simulink model "UAM_FlightMode"  (R2024b)
settings: Solver=FixedStepAuto  StartTime=0.0  StopTime=10.0  RelTol=1e-3
model workspace: external: MAT-File C:\Users\admin\Desktop\onboard-flight-control-software-ver1.1\data\stateBus.mat (data not in the file)
undefined symbols (not defined in the file): control, FSState, Vt, zGround
libraries: uavalgslib x6, simulink x1
settings Model: DataDictionary=UAM_data.sldd  Creator=admin  LastModifiedBy=admin
settings OptimizationCC: DefaultParameterBehavior=Inlined  EnhancedBackFolding=on  PassReuseOutputArgsAs=Individual arguments  ZeroExternalMemoryAtStartup=off  ZeroInternalMemoryAtStartup=off  OptimizeBlockOrder=speed  DifferentSizesBufferReuse=on  OptimizationCustomize=off  EfficientTunableParamExpr=on
settings DebuggingCC: ParameterTunabilityLossMsg=error
settings HardwareCC: ProdBitPerLong=64  ProdLargestAtomicInteger=LongLong  ProdLargestAtomicFloat=Double  ProdLongLongMode=on  ProdHWDeviceType=ARM Compatible->ARM Cortex-A (64-bit)
settings SFSimCC: MATLABDynamicMemAlloc=off
settings RTWCC: Description=Embedded Coder  SystemTargetFile=ert.tlc  TemplateMakefile=ert_default_tmf  Toolchain=Linaro AArch64 Linux v6.3.1
settings CodeAppCC: ForceParamTrailComments=on  IgnoreCustomStorageClasses=off  OperatorAnnotations=on  SimulinkDataObjDesc=on  SFDataObjDesc=on  CustomSymbolStrGlobalVar=MODE_$N$M  CustomSymbolStrType=MODE_$N$M_T  CustomSymbolStrField=MODE_$N$M  CustomSymbolStrFcn=MODE_$N$M$F  CustomSymbolStrBlkIO=MODE_rtb_$N$M  CustomSymbolStrTmpVar=MODE_tmp_$N$M  CustomSymbolStrMacro=MODE_$N$M_MACRO  InsertBlockDesc=on
settings ERTTargetCC: TargetLangStandard=C99 (ISO)  GenerateSampleERTMain=on  ERTCustomFileTemplate=example_file_process.tlc

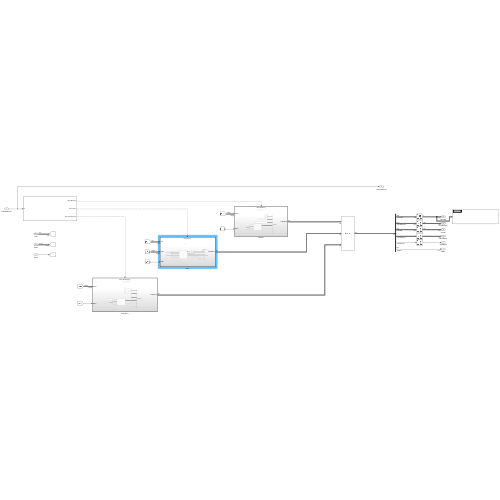
[thumbnail: Simulink's stored preview of the top-level diagram]
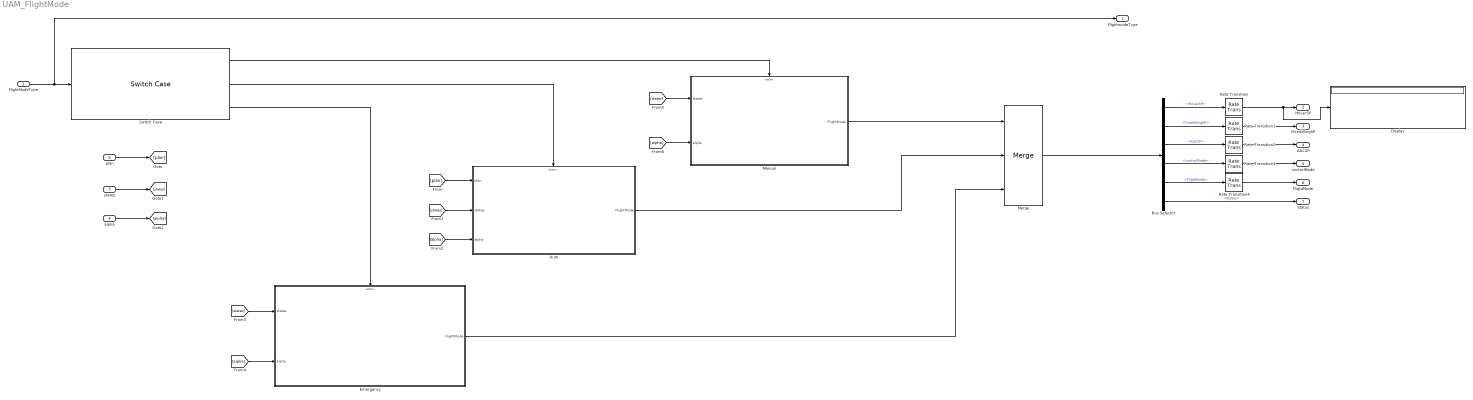
== system UAM_FlightMode ==
  FlightModeType : Inport
  plan : Inport  Port=2  OutDataTypeStr=Bus: plan
  states : Inport  Port=3  OutDataTypeStr=Bus: states
  alpha : Inport  Port=4
  Auto : Subsystem  TreatAsAtomicUnit=on
  Bus Selector : BusSelector  OutputSignals=HoverSP,FixedWingSP,AACSP,controlMode,FlightMode,Status
  Display : Display
  Emergency : Subsystem  TreatAsAtomicUnit=on
  Manual : Subsystem  TreatAsAtomicUnit=on
  Merge : Merge  Inputs=3
  Rate Transition{,1..4} (5 alike) : RateTransition
  Switch Case : SwitchCase  CaseConditions={FlightModeType.Manual, FlightModeType.Auto, FlightModeType.Emergecny}  ShowDefaultCase=off
  FlightmodeType : Outport  OutDataTypeStr=Enum: FlightModeType
  HoverSP : Outport  Port=2  OutDataTypeStr=Bus: HoverSPBus
  FixedWingSP : Outport  Port=3  OutDataTypeStr=Bus: FixedWingCommandBus
  AACSP : Outport  Port=4  OutDataTypeStr=Bus: AAC
  controlMode : Outport  Port=5  OutDataTypeStr=Bus: controlMode
  FlightMode : Outport  Port=6
  Status : Outport  Port=7
  wires:
  FlightModeType/1 -> FlightmodeType/1, Switch Case/1
  plan/1 -> [plan]
  states/1 -> [states]
  [states] -> Auto/2(states)
  [alpha] -> Auto/3(alpha)
  alpha/1 -> [alpha]
  [plan] -> Auto/1(plan)
  Switch Case/2 -> Auto/Action
  Switch Case/1 -> Manual/Action
  Switch Case/3 -> Emergency/Action
  [alpha] -> Emergency/2(alpha)
  [states] -> Emergency/1(states)
  [alpha] -> Manual/2(alpha)
  [states] -> Manual/1(states)
  Manual/1(FlightMode) -> Merge/1
  Bus Selector/4 -> Rate Transition3/1  "<controlMode>"
  Rate Transition1/1 -> FixedWingSP/1
  Bus Selector/5 -> Rate Transition4/1  "<FlightMode>"
  Rate Transition3/1 -> controlMode/1
  Bus Selector/1 -> Rate Transition/1  "<HoverSP>"
  Bus Selector/3 -> Rate Transition2/1  "<AACSP>"
  Rate Transition/1 -> Display/1, HoverSP/1
  Rate Transition4/1 -> FlightMode/1
  Bus Selector/2 -> Rate Transition1/1  "<FixedWingSP>"
  Rate Transition2/1 -> AACSP/1
  Bus Selector/6 -> Status/1  "<Status>"
  Merge/1 -> Bus Selector/1
  Auto/1(FlightMode) -> Merge/2
  Emergency/1(FlightMode) -> Merge/3

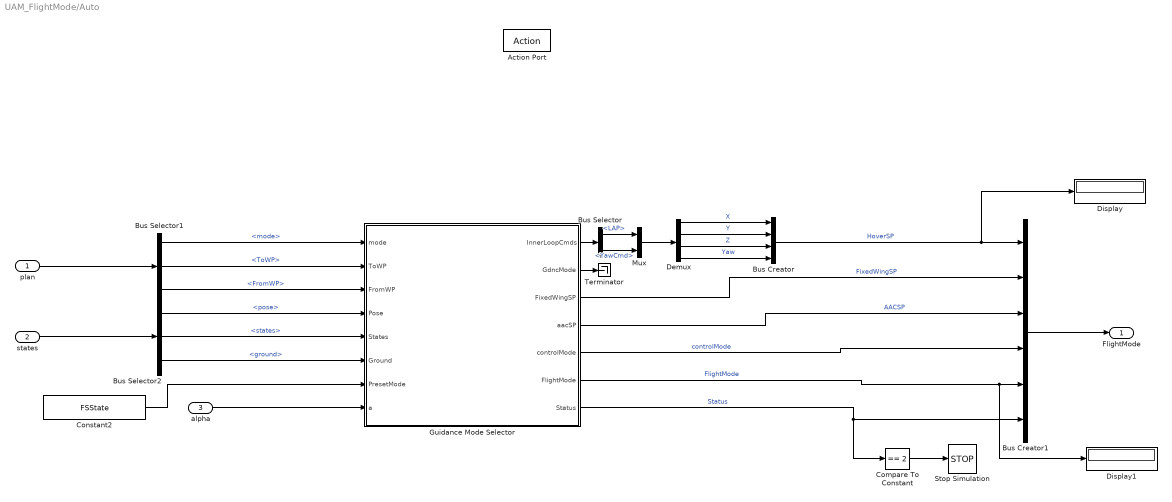
== system UAM_FlightMode/Auto ==
  plan : Inport  OutDataTypeStr=Bus: plan
  states : Inport  Port=2  OutDataTypeStr=Bus: states
  alpha : Inport  Port=3
  Action Port : ActionPort  ActionPortLabel=case [ Auto ]:
  Bus Creator : BusCreator  Inputs=4  OutDataTypeStr=Bus: HoverSPBus
      settings: InheritFromInputs=off
  Bus Creator1 : BusCreator  Inputs=6  OutDataTypeStr=Bus: flightmode
  Bus Selector : BusSelector  OutputSignals=LAP,YawCmd
  Bus Selector1 : BusSelector  OutputSignals=mode,ToWP,FromWP
  Bus Selector2 : BusSelector  OutputSignals=pose,states,ground
  Compare To Constant : simulink/Logic and Bit Operations/Compare To Constant  relop===  const=2  OutDataTypeStr=boolean
  Constant2 : Constant  Value=FSState
  Demux : Demux
  Display : Display
  Display1 : Display
  Guidance Mode Selector : Stateflow chart  TreatAsAtomicUnit=on
      settings: PortSchema="{\"entries\":[{\"content\":{\"sides\":[{\"content\":{\"connectorIds\":[\"In1\",\"In2\",\"In3\",\"In4\",\"In5\",\"In7\",\"In6\",\"In8\"]},\"type\":\"ConnectorPlacement.EquallySpacedRectSide\",\"uuid\":\"a9cfd0e2-196c-422d-b359-9161a47768c9\"},{\"content\":{\"connectorIds\":[\"Out7\",\"Out2\",\"Out4\",\"Out3\",\"Out5\",\"Out6\",\"Out1\"],\"side\":\"RIGHT\"},\"type\":\"ConnectorPlacement.EquallySpacedRectSide\",\"uuid\":\"4fed41ae-e7cf-4de3-8bdb-9e24e7d8b079\"},{\"content\":{\"side\":\"TOP\"},\"type\":\"ConnectorPlacement.EquallySpacedRectSide\",\"uuid\":\"2d49ff20-2f63-498d-ac9d-820eae01f794\"},{\"content\":{\"side\":\"BOTTOM\"},\"type\":\"ConnectorPlacement.EquallySpacedRectSide\",\"uuid\":\"da24ee44-6e15-4e50-9b36-ff21cb47946d\"}]},\"type\":\"ConnectorPlacement.EquallySpacedConnector\",\"uuid\":\"88d403f4-ad96-40f9-9697-84906f26a8bf\"}],\"packageUris\":[\"http://schema.mathworks.com/mf0/Connector/R2020b\"],\"version\":\"1.0\"}"
  Mux : Mux  Inputs=2
  Stop Simulation : Stop
  Terminator : Terminator
  FlightMode : Outport  OutDataTypeStr=Bus: flightmode
  wires:
  Bus Selector1/1 -> Guidance Mode Selector/1(mode)  "<mode>"
  Guidance Mode Selector/6(FlightMode) -> Display1/1, Bus Creator1/5  "FlightMode"
  Bus Selector1/3 -> Guidance Mode Selector/3(FromWP)  "<FromWP>"
  Bus Selector2/3 -> Guidance Mode Selector/7(Ground)  "<ground>"
  Bus Selector/1 -> Mux/1  "<LAP>"
  Guidance Mode Selector/5(controlMode) -> Bus Creator1/4  "controlMode"
  Guidance Mode Selector/3(aacSP) -> Bus Creator1/3  "AACSP"
  alpha/1 -> Guidance Mode Selector/8(a)
  Guidance Mode Selector/7(InnerLoopCmds) -> Bus Selector/1
  Guidance Mode Selector/2(GdncMode) -> Terminator/1
  Bus Selector/2 -> Mux/2  "<YawCmd>"
  Compare To Constant/1 -> Stop Simulation/1
  Bus Selector2/2 -> Guidance Mode Selector/5(States)  "<states>"
  Mux/1 -> Demux/1
  plan/1 -> Bus Selector1/1
  states/1 -> Bus Selector2/1
  Bus Selector2/1 -> Guidance Mode Selector/4(Pose)  "<pose>"
  Guidance Mode Selector/1(Status) -> Compare To Constant/1, Bus Creator1/6  "Status"
  Guidance Mode Selector/4(FixedWingSP) -> Bus Creator1/2  "FixedWingSP"
  Constant2/1 -> Guidance Mode Selector/6(PresetMode)
  Bus Selector1/2 -> Guidance Mode Selector/2(ToWP)  "<ToWP>"
  Bus Creator1/1 -> FlightMode/1
  Demux/1 -> Bus Creator/1  "X"
  Demux/2 -> Bus Creator/2  "Y"
  Demux/3 -> Bus Creator/3  "Z"
  Demux/4 -> Bus Creator/4  "Yaw"
  Bus Creator/1 -> Display/1, Bus Creator1/1  "HoverSP"

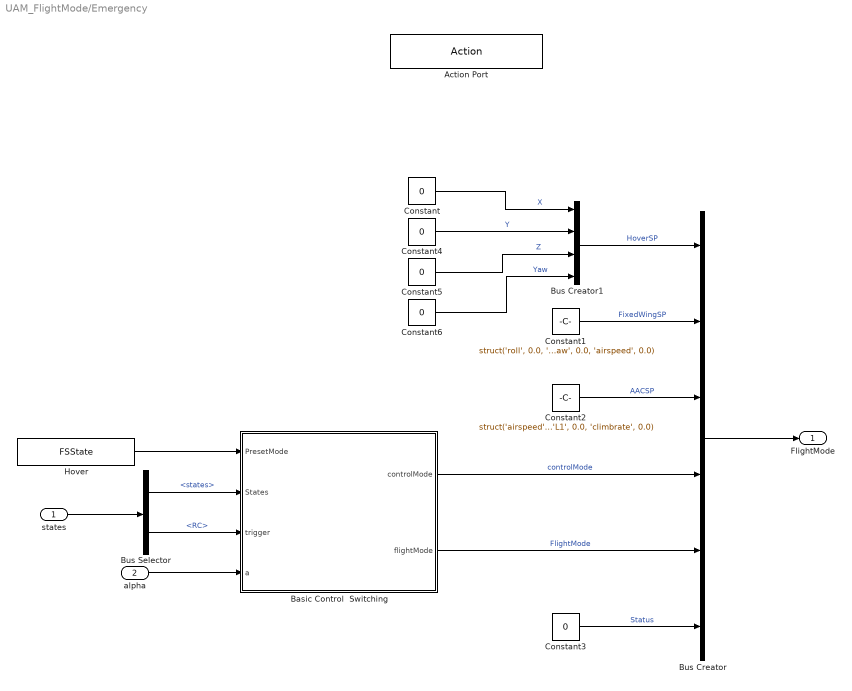
== system UAM_FlightMode/Emergency ==
  states : Inport  OutDataTypeStr=Bus: states
  alpha : Inport  Port=2
  Action Port : ActionPort  ActionPortLabel=case [ Emergecny ]:
  Basic Control  Switching : Stateflow chart  TreatAsAtomicUnit=on
  Bus Creator : BusCreator  Inputs=6  OutDataTypeStr=Bus: flightmode
      settings: InheritFromInputs=off
  Bus Creator1 : BusCreator  Inputs=4  OutDataTypeStr=Bus: HoverSPBus
  Bus Selector : BusSelector  OutputSignals=states,states.RC
  Constant{,4..6} (4 alike) : Constant  Value=0
  Constant1 : Constant  Value=struct('roll', 0.0, 'pitch', 0.0, 'yaw', 0.0, 'airspeed', 0.0)  VectorParams1D=off  OutDataTypeStr=Bus: FixedWingCommandBus
  Constant2 : Constant  Value=struct('airspeed', 0.0, 'altitude', 0.0, 'course', 0.0, 'L1', 0.0, 'climbrate', 0.0)  VectorParams1D=off  OutDataTypeStr=Bus: AAC
  Constant3 : Constant  Value=0  OutDataTypeStr=uint8
  Hover : Constant  Value=FSState
  FlightMode : Outport  OutDataTypeStr=Bus: flightmode
  wires:
  Constant/1 -> Bus Creator1/1  "X"
  Constant5/1 -> Bus Creator1/3  "Z"
  Constant4/1 -> Bus Creator1/2  "Y"
  Basic Control  Switching/2(flightMode) -> Bus Creator/5  "FlightMode"
  Basic Control  Switching/1(controlMode) -> Bus Creator/4  "controlMode"
  Hover/1 -> Basic Control  Switching/1(PresetMode)
  Constant3/1 -> Bus Creator/6  "Status"
  Bus Selector/2 -> Basic Control  Switching/3(trigger)  "<RC>"
  Bus Selector/1 -> Basic Control  Switching/2(States)  "<states>"
  Constant2/1 -> Bus Creator/3  "AACSP"
  alpha/1 -> Basic Control  Switching/4(a)
  Bus Creator1/1 -> Bus Creator/1  "HoverSP"
  states/1 -> Bus Selector/1
  Constant1/1 -> Bus Creator/2  "FixedWingSP"
  Constant6/1 -> Bus Creator1/4  "Yaw"
  Bus Creator/1 -> FlightMode/1

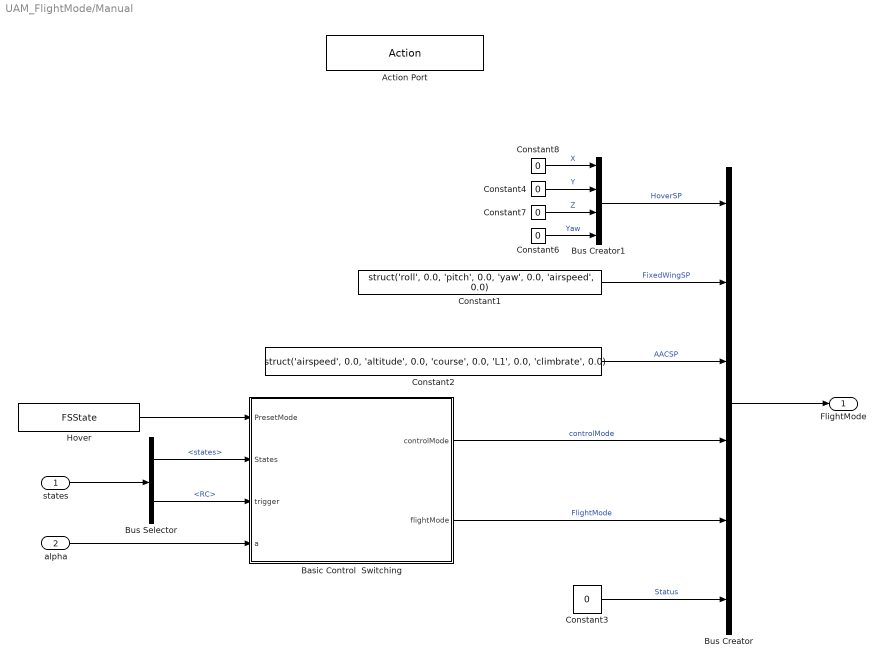
== system UAM_FlightMode/Manual ==
  states : Inport  OutDataTypeStr=Bus: states
  alpha : Inport  Port=2
  Action Port : ActionPort  ActionPortLabel=case [ Manual ]:
  Basic Control  Switching : Stateflow chart  TreatAsAtomicUnit=on
  Bus Creator : BusCreator  Inputs=6  OutDataTypeStr=Bus: flightmode
      settings: InheritFromInputs=off
  Bus Creator1 : BusCreator  Inputs=4  OutDataTypeStr=Bus: HoverSPBus
  Bus Selector : BusSelector  OutputSignals=states,states.RC
  Constant1 : Constant  Value=struct('roll', 0.0, 'pitch', 0.0, 'yaw', 0.0, 'airspeed', 0.0)  VectorParams1D=off  OutDataTypeStr=Bus: FixedWingCommandBus
  Constant2 : Constant  Value=struct('airspeed', 0.0, 'altitude', 0.0, 'course', 0.0, 'L1', 0.0, 'climbrate', 0.0)  VectorParams1D=off  OutDataTypeStr=Bus: AAC
  Constant3 : Constant  Value=0  OutDataTypeStr=uint8
  Constant{4,6..8} (4 alike) : Constant  Value=0
  Hover : Constant  Value=FSState
  FlightMode : Outport  OutDataTypeStr=Bus: flightmode
  wires:
  states/1 -> Bus Selector/1
  Basic Control  Switching/1(controlMode) -> Bus Creator/4  "controlMode"
  Hover/1 -> Basic Control  Switching/1(PresetMode)
  Basic Control  Switching/2(flightMode) -> Bus Creator/5  "FlightMode"
  Constant3/1 -> Bus Creator/6  "Status"
  Bus Creator/1 -> FlightMode/1
  Bus Creator1/1 -> Bus Creator/1  "HoverSP"
  Constant2/1 -> Bus Creator/3  "AACSP"
  Constant1/1 -> Bus Creator/2  "FixedWingSP"
  alpha/1 -> Basic Control  Switching/4(a)
  Bus Selector/1 -> Basic Control  Switching/2(States)  "<states>"
  Bus Selector/2 -> Basic Control  Switching/3(trigger)  "<RC>"
  Constant6/1 -> Bus Creator1/4  "Yaw"
  Constant7/1 -> Bus Creator1/3  "Z"
  Constant4/1 -> Bus Creator1/2  "Y"
  Constant8/1 -> Bus Creator1/1  "X"

== system UAM_FlightMode/Auto/Guidance Mode Selector/GuidanceLogic.BackTransition ==
  States : Inport  OutDataTypeStr=Bus: GuidanceStates
  Action Port : ActionPort
      settings: CopyFcn=Stateflow.SLINSF.SimulinkMan.removeBlockPreDeleteFcn  PreDeleteFcn=Stateflow.SLINSF.SimulinkMan.unsafePredeleteFcn
  Bus Creator1 : BusCreator  Inputs=3  OutDataTypeStr=Bus: innerLoopCmdsBus  NonVirtualBus=on
  Bus Selector : BusSelector  OutputSignals=Xe
  Constant : Constant  Value=0
  Constant1 : Constant  Value=0
  Constant2 : Constant  Value=0
  Data Type Conversion : DataTypeConversion  OutDataTypeStr=uint8  SaturateOnIntegerOverflow=off  RndMeth=Floor
  Gain : Gain
  Status : Outport
  InnerLoopCmds : Outport  Port=2  OutDataTypeStr=Bus: innerLoopCmdsBus
  wires:
  States/1 -> Bus Selector/1
  Bus Selector/1 -> Gain/1  "<Xe>"
  Bus Creator1/1 -> InnerLoopCmds/1
  Constant1/1 -> Bus Creator1/2  "HeadingCmd"
  Constant2/1 -> Bus Creator1/3  "YawCmd"
  Data Type Conversion/1 -> Status/1
  Gain/1 -> Bus Creator1/1  "LAP"
  Constant/1 -> Data Type Conversion/1

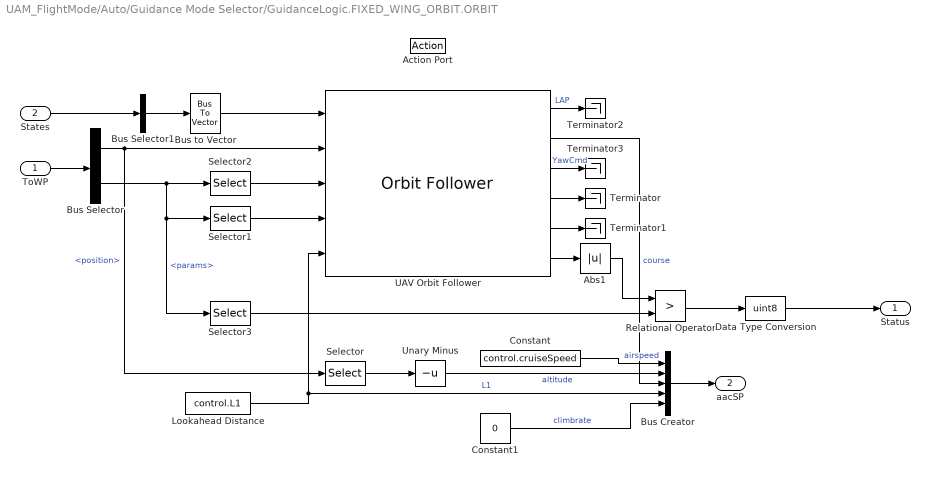
== system UAM_FlightMode/Auto/Guidance Mode Selector/GuidanceLogic.FIXED_WING_ORBIT.ORBIT ==
  ToWP : Inport  OutDataTypeStr=Bus: UAVPathManagerBus
  States : Inport  Port=2
  Action Port : ActionPort
      settings: CopyFcn=Stateflow.SLINSF.SimulinkMan.removeBlockPreDeleteFcn  PreDeleteFcn=Stateflow.SLINSF.SimulinkMan.unsafePredeleteFcn
  Abs1 : Abs  SaturateOnIntegerOverflow=off
  Bus Creator : BusCreator  Inputs=5  OutDataTypeStr=Bus: AAC  NonVirtualBus=on
      settings: InheritFromInputs=off
  Bus Selector : BusSelector  OutputSignals=position,params
  Bus Selector1 : BusSelector  OutputSignals=Xe,course  OutputAsBus=on
  Bus to Vector : BusToVector
  Constant : Constant  Value=control.cruiseSpeed
  Constant1 : Constant  Value=0
  Data Type Conversion : DataTypeConversion  OutDataTypeStr=uint8  SaturateOnIntegerOverflow=off  RndMeth=Floor
  Lookahead Distance : Constant  Value=control.L1  OutDataTypeStr=double
  Relational Operator : RelationalOperator  Operator=>  OutDataTypeStr=boolean  RndMeth=Simplest  InputSameDT=off
  Selector : Selector  InputPortWidth=3  IndexOptions=Index vector (dialog)  Indices=3  OutputSizes=1
  Selector1 : Selector  InputPortWidth=4  IndexOptions=Index vector (dialog)  Indices=2  OutputSizes=1
  Selector2 : Selector  InputPortWidth=4  IndexOptions=Index vector (dialog)  Indices=1  OutputSizes=1
  Selector3 : Selector  InputPortWidth=4  IndexOptions=Index vector (dialog)  Indices=3  OutputSizes=1
  Terminator{,1..3} (4 alike) : Terminator
  UAV Orbit Follower : uavalgslib/Orbit Follower  UAVType=fixed-wing  MinOrbitRadius=control.turningRadius  MinLookaheadDistance=control.L1  ExternalReset=none  ShowCrossTrackErrorOutput=off  ShowNumTurnsOutput=on  SimulateUsing=Code generation
  Unary Minus : UnaryMinus
  Status : Outport
  aacSP : Outport  Port=2
  wires:
  Bus to Vector/1 -> UAV Orbit Follower/1
  Selector2/1 -> UAV Orbit Follower/3
  Bus Selector/1 -> UAV Orbit Follower/2, Selector/1  "<position>"
  ToWP/1 -> Bus Selector/1
  Bus Selector/2 -> Selector1/1, Selector3/1, Selector2/1  "<params>"
  Selector3/1 -> Relational Operator/2
  Relational Operator/1 -> Data Type Conversion/1
  UAV Orbit Follower/4 -> Terminator/1
  UAV Orbit Follower/5 -> Terminator1/1
  Bus Selector1/1 -> Bus to Vector/1
  States/1 -> Bus Selector1/1
  UAV Orbit Follower/1 -> Terminator2/1  "LAP"
  Lookahead Distance/1 -> UAV Orbit Follower/5, Bus Creator/4  "L1"
  Bus Creator/1 -> aacSP/1
  UAV Orbit Follower/2 -> Bus Creator/3  "course"
  Constant/1 -> Bus Creator/1  "airspeed"
  Unary Minus/1 -> Bus Creator/2  "altitude"
  UAV Orbit Follower/3 -> Terminator3/1  "YawCmd"
  Selector/1 -> Unary Minus/1
  UAV Orbit Follower/6 -> Abs1/1
  Abs1/1 -> Relational Operator/1
  Selector1/1 -> UAV Orbit Follower/4
  Constant1/1 -> Bus Creator/5  "climbrate"
  Data Type Conversion/1 -> Status/1

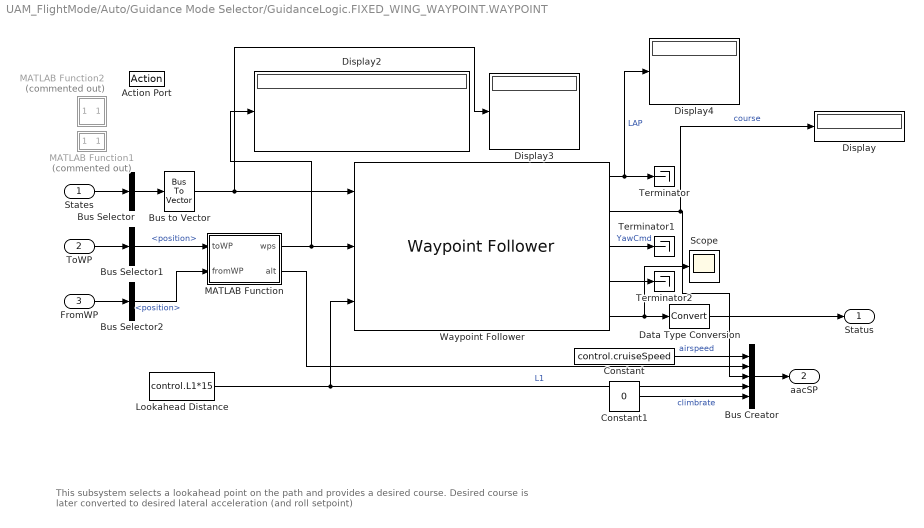
== system UAM_FlightMode/Auto/Guidance Mode Selector/GuidanceLogic.FIXED_WING_WAYPOINT.WAYPOINT ==
  note: This subsystem selects a lookahead point on the path and provides a desired course. Desired course is later converted to desired lateral acceleration (and roll setpoint)
  States : Inport  OutDataTypeStr=Bus: GuidanceStates
  ToWP : Inport  Port=2  OutDataTypeStr=Bus: UAVPathManagerBus
  FromWP : Inport  Port=3  OutDataTypeStr=Bus: UAVPathManagerBus
  Action Port : ActionPort
      settings: CopyFcn=Stateflow.SLINSF.SimulinkMan.removeBlockPreDeleteFcn  PreDeleteFcn=Stateflow.SLINSF.SimulinkMan.unsafePredeleteFcn
  Bus Creator : BusCreator  Inputs=5  OutDataTypeStr=Bus: AAC  NonVirtualBus=on
      settings: InheritFromInputs=off
  Bus Selector : BusSelector  OutputSignals=Xe,course  OutputAsBus=on
  Bus Selector1 : BusSelector  OutputSignals=position
  Bus Selector2 : BusSelector  OutputSignals=position
  Bus to Vector : BusToVector
  Constant : Constant  Value=control.cruiseSpeed
  Constant1 : Constant  Value=0
  Data Type Conversion : DataTypeConversion  SaturateOnIntegerOverflow=off  RndMeth=Floor
  Display{,2..4} (4 alike) : Display
  Lookahead Distance : Constant  Value=control.L1*15  OutDataTypeStr=double
  MATLAB Function : MATLAB Function  TreatAsAtomicUnit=on
  MATLAB Function1 : MATLAB Function  Commented=on  TreatAsAtomicUnit=on
  MATLAB Function2 : MATLAB Function  Commented=on  TreatAsAtomicUnit=on
  Scope : Scope
  Terminator : Terminator
  Terminator1 : Terminator
  Terminator2 : Terminator
  Waypoint Follower : uavalgslib/Waypoint Follower  UAVType=fixed-wing  StartFrom=first  TransitionRadiusSource=internal  TransitionRadius=FWControl.transitionRadius  MinLookaheadDistance=control.L1  HoverAtLastWaypoint=off  YawInput=off  ShowCrossTrackErrorOutput=off  ShowStatusOutput=on  SimulateUsing=Code generation
  Status : Outport
  aacSP : Outport  Port=2
  wires:
  Lookahead Distance/1 -> Waypoint Follower/3, Bus Creator/4  "L1"
  Waypoint Follower/1 -> Display4/1, Terminator/1  "LAP"
  Waypoint Follower/3 -> Terminator1/1  "YawCmd"
  Waypoint Follower/4 -> Terminator2/1
  Constant/1 -> Bus Creator/1  "airspeed"
  States/1 -> Bus Selector/1
  Bus Selector/1 -> Bus to Vector/1
  Waypoint Follower/5 -> Scope/1, Data Type Conversion/1
  Data Type Conversion/1 -> Status/1
  Bus Creator/1 -> aacSP/1
  ToWP/1 -> Bus Selector1/1
  FromWP/1 -> Bus Selector2/1
  Bus Selector1/1 -> MATLAB Function/1(toWP)  "<position>"
  Bus Selector2/1 -> MATLAB Function/2(fromWP)  "<position>"
  MATLAB Function/2(alt) -> Bus Creator/2
  Waypoint Follower/2 -> Display/1, Bus Creator/3  "course"
  Constant1/1 -> Bus Creator/5  "climbrate"
  Bus to Vector/1 -> Display3/1, Waypoint Follower/1
  MATLAB Function/1(wps) -> Display2/1, Waypoint Follower/2

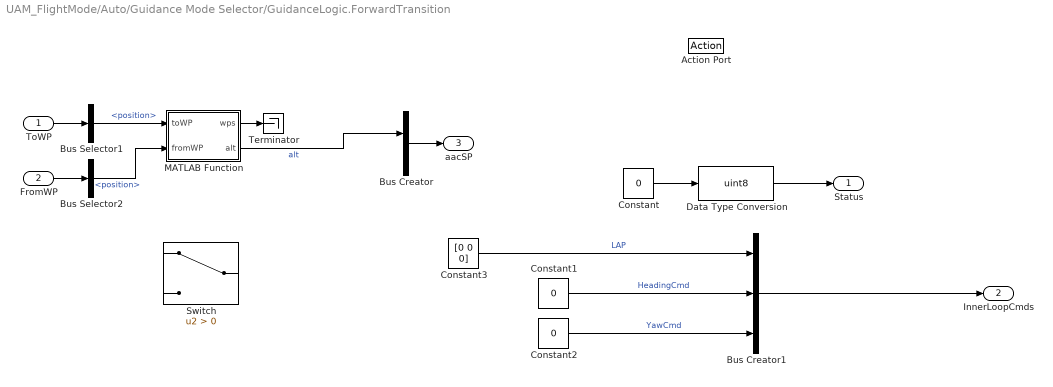
== system UAM_FlightMode/Auto/Guidance Mode Selector/GuidanceLogic.ForwardTransition ==
  ToWP : Inport  OutDataTypeStr=Bus: UAVPathManagerBus
  FromWP : Inport  Port=2  OutDataTypeStr=Bus: UAVPathManagerBus
  Action Port : ActionPort
      settings: CopyFcn=Stateflow.SLINSF.SimulinkMan.removeBlockPreDeleteFcn  PreDeleteFcn=Stateflow.SLINSF.SimulinkMan.unsafePredeleteFcn
  Bus Creator : BusCreator  Inputs=5  OutDataTypeStr=Bus: AAC  NonVirtualBus=on
      settings: InheritFromInputs=off
  Bus Creator1 : BusCreator  Inputs=3  OutDataTypeStr=Bus: innerLoopCmdsBus  NonVirtualBus=on
  Bus Selector1 : BusSelector  OutputSignals=position
  Bus Selector2 : BusSelector  OutputSignals=position
  Constant : Constant  Value=0
  Constant1 : Constant  Value=0
  Constant2 : Constant  Value=0
  Constant3 : Constant  Value=[0 0 0]
  Data Type Conversion : DataTypeConversion  OutDataTypeStr=uint8  SaturateOnIntegerOverflow=off  RndMeth=Floor
  MATLAB Function : MATLAB Function  TreatAsAtomicUnit=on
  Switch : Switch  Criteria=u2 > Threshold  SaturateOnIntegerOverflow=off  InputSameDT=off
  Terminator : Terminator
  Status : Outport
  InnerLoopCmds : Outport  Port=2  OutDataTypeStr=Bus: innerLoopCmdsBus
  aacSP : Outport  Port=3
  wires:
  Bus Creator1/1 -> InnerLoopCmds/1
  Constant1/1 -> Bus Creator1/2  "HeadingCmd"
  Constant2/1 -> Bus Creator1/3  "YawCmd"
  Data Type Conversion/1 -> Status/1
  Constant/1 -> Data Type Conversion/1
  Constant3/1 -> Bus Creator1/1  "LAP"
  FromWP/1 -> Bus Selector2/1
  Bus Selector1/1 -> MATLAB Function/1(toWP)  "<position>"
  Bus Selector2/1 -> MATLAB Function/2(fromWP)  "<position>"
  ToWP/1 -> Bus Selector1/1
  Bus Creator/1 -> aacSP/1
  MATLAB Function/1(wps) -> Terminator/1
  MATLAB Function/2(alt) -> Bus Creator/2  "alt"

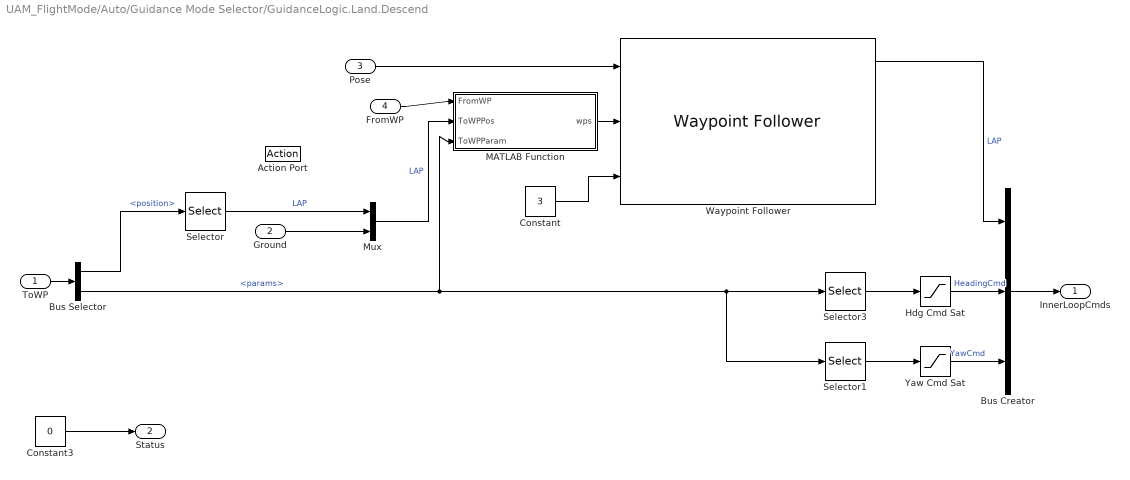
== system UAM_FlightMode/Auto/Guidance Mode Selector/GuidanceLogic.Land.Descend ==
  ToWP : Inport  OutDataTypeStr=Bus: UAVPathManagerBus
  Ground : Inport  Port=2
  Pose : Inport  Port=3
  FromWP : Inport  Port=4  OutDataTypeStr=Bus: UAVPathManagerBus
  Action Port : ActionPort
      settings: CopyFcn=Stateflow.SLINSF.SimulinkMan.removeBlockPreDeleteFcn  PreDeleteFcn=Stateflow.SLINSF.SimulinkMan.unsafePredeleteFcn
  Bus Creator : BusCreator  Inputs=3  OutDataTypeStr=Bus: innerLoopCmdsBus  NonVirtualBus=on
      settings: InheritFromInputs=off
  Bus Selector : BusSelector  OutputSignals=position,params
  Constant : Constant  Value=3
  Constant3 : Constant  Value=0  OutDataTypeStr=uint8
  Hdg Cmd Sat : Saturate  UpperLimit=pi  LowerLimit=-pi
      settings: AttributesFormatString=[%<UpperLimit> %<LowerLimit>]
  MATLAB Function : MATLAB Function  TreatAsAtomicUnit=on
  Mux : Mux  Inputs=2
  Selector : Selector  InputPortWidth=3  IndexOptions=Index vector (dialog)  Indices=[1 2]  OutputSizes=1
  Selector1 : Selector  InputPortWidth=4  IndexOptions=Index vector (dialog)  Indices=4  OutputSizes=1
  Selector3 : Selector  InputPortWidth=4  IndexOptions=Index vector (dialog)  Indices=4  OutputSizes=1
  Waypoint Follower : uavalgslib/Waypoint Follower  UAVType=multirotor  StartFrom=first  TransitionRadiusSource=internal  TransitionRadius=1  MinLookaheadDistance=0.1  HoverAtLastWaypoint=on  YawInput=on  ShowCrossTrackErrorOutput=off  ShowStatusOutput=off  SimulateUsing=Code generation
  Yaw Cmd Sat : Saturate  UpperLimit=pi  LowerLimit=-pi
      settings: AttributesFormatString=[%<UpperLimit> %<LowerLimit>]
  InnerLoopCmds : Outport  OutDataTypeStr=Bus: innerLoopCmdsBus
  Status : Outport  Port=2
  wires:
  Bus Creator/1 -> InnerLoopCmds/1
  Bus Selector/1 -> Selector/1  "<position>"
  Yaw Cmd Sat/1 -> Bus Creator/3  "YawCmd"
  Hdg Cmd Sat/1 -> Bus Creator/2  "HeadingCmd"
  ToWP/1 -> Bus Selector/1
  Selector1/1 -> Yaw Cmd Sat/1
  Selector3/1 -> Hdg Cmd Sat/1
  Selector/1 -> Mux/1  "LAP"
  Bus Selector/2 -> MATLAB Function/3(ToWPParam), Selector1/1, Selector3/1  "<params>"
  Ground/1 -> Mux/2
  Constant3/1 -> Status/1
  Mux/1 -> MATLAB Function/2(ToWPPos)  "LAP"
  FromWP/1 -> MATLAB Function/1(FromWP)
  Pose/1 -> Waypoint Follower/1
  MATLAB Function/1(wps) -> Waypoint Follower/2
  Constant/1 -> Waypoint Follower/3
  Waypoint Follower/1 -> Bus Creator/1  "LAP"

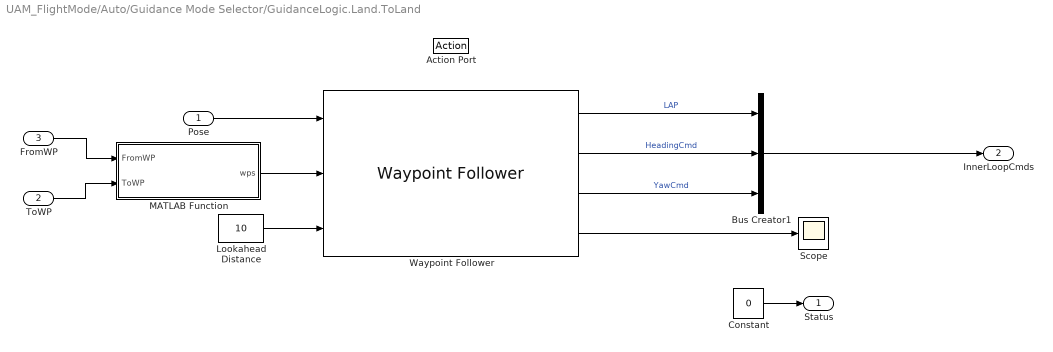
== system UAM_FlightMode/Auto/Guidance Mode Selector/GuidanceLogic.Land.ToLand ==
  Pose : Inport
  ToWP : Inport  Port=2  OutDataTypeStr=Bus: UAVPathManagerBus
  FromWP : Inport  Port=3  OutDataTypeStr=Bus: UAVPathManagerBus
  Action Port : ActionPort
      settings: CopyFcn=Stateflow.SLINSF.SimulinkMan.removeBlockPreDeleteFcn  PreDeleteFcn=Stateflow.SLINSF.SimulinkMan.unsafePredeleteFcn
  Bus Creator1 : BusCreator  Inputs=3  OutDataTypeStr=Bus: innerLoopCmdsBus  NonVirtualBus=on
  Constant : Constant  Value=0  OutDataTypeStr=uint8
  Lookahead Distance : Constant  Value=10  OutDataTypeStr=double
  MATLAB Function : MATLAB Function  TreatAsAtomicUnit=on
  Scope : Scope
  Waypoint Follower : uavalgslib/Waypoint Follower  UAVType=multirotor  StartFrom=first  TransitionRadiusSource=internal  TransitionRadius=1  MinLookaheadDistance=0.1  HoverAtLastWaypoint=on  YawInput=on  ShowCrossTrackErrorOutput=off  ShowStatusOutput=off  SimulateUsing=Code generation
  Status : Outport
  InnerLoopCmds : Outport  Port=2  OutDataTypeStr=Bus: innerLoopCmdsBus
  wires:
  Constant/1 -> Status/1
  MATLAB Function/1(wps) -> Waypoint Follower/2
  Lookahead Distance/1 -> Waypoint Follower/3
  Bus Creator1/1 -> InnerLoopCmds/1
  ToWP/1 -> MATLAB Function/2(ToWP)
  Waypoint Follower/2 -> Bus Creator1/2  "HeadingCmd"
  FromWP/1 -> MATLAB Function/1(FromWP)
  Waypoint Follower/4 -> Scope/1
  Pose/1 -> Waypoint Follower/1
  Waypoint Follower/3 -> Bus Creator1/3  "YawCmd"
  Waypoint Follower/1 -> Bus Creator1/1  "LAP"

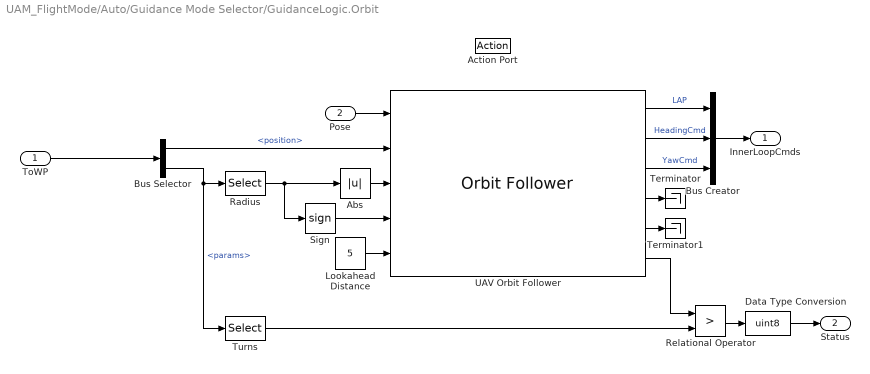
== system UAM_FlightMode/Auto/Guidance Mode Selector/GuidanceLogic.Orbit ==
  ToWP : Inport  OutDataTypeStr=Bus: UAVPathManagerBus
  Pose : Inport  Port=2
  Action Port : ActionPort
      settings: CopyFcn=Stateflow.SLINSF.SimulinkMan.removeBlockPreDeleteFcn  PreDeleteFcn=Stateflow.SLINSF.SimulinkMan.unsafePredeleteFcn
  Abs : Abs  SaturateOnIntegerOverflow=off
  Bus Creator : BusCreator  Inputs=3  OutDataTypeStr=Bus: innerLoopCmdsBus  NonVirtualBus=on
  Bus Selector : BusSelector  OutputSignals=position,params
  Data Type Conversion : DataTypeConversion  OutDataTypeStr=uint8  SaturateOnIntegerOverflow=off  RndMeth=Floor
  Lookahead Distance : Constant  Value=5  OutDataTypeStr=double
  Radius : Selector  InputPortWidth=4  IndexOptions=Index vector (dialog)  Indices=[3]  OutputSizes=1
  Relational Operator : RelationalOperator  Operator=>  OutDataTypeStr=boolean  RndMeth=Simplest  InputSameDT=off
  Sign : Signum  ZeroCross=off
  Terminator : Terminator
  Terminator1 : Terminator
  Turns : Selector  InputPortWidth=4  IndexOptions=Index vector (dialog)  Indices=[1]  OutputSizes=1
  UAV Orbit Follower : uavalgslib/Orbit Follower  UAVType=multirotor  MinOrbitRadius=1  MinLookaheadDistance=0.1  ExternalReset=none  ShowCrossTrackErrorOutput=off  ShowNumTurnsOutput=on  SimulateUsing=Code generation
  InnerLoopCmds : Outport  OutDataTypeStr=Bus: innerLoopCmdsBus
  Status : Outport  Port=2
  wires:
  Pose/1 -> UAV Orbit Follower/1
  Lookahead Distance/1 -> UAV Orbit Follower/5
  Abs/1 -> UAV Orbit Follower/3
  Bus Selector/1 -> UAV Orbit Follower/2  "<position>"
  ToWP/1 -> Bus Selector/1
  Bus Creator/1 -> InnerLoopCmds/1
  UAV Orbit Follower/2 -> Bus Creator/2  "HeadingCmd"
  UAV Orbit Follower/3 -> Bus Creator/3  "YawCmd"
  Bus Selector/2 -> Turns/1, Radius/1  "<params>"
  Radius/1 -> Abs/1, Sign/1
  Sign/1 -> UAV Orbit Follower/4
  Relational Operator/1 -> Data Type Conversion/1
  Turns/1 -> Relational Operator/2
  Data Type Conversion/1 -> Status/1
  UAV Orbit Follower/6 -> Relational Operator/1
  UAV Orbit Follower/4 -> Terminator/1
  UAV Orbit Follower/5 -> Terminator1/1
  UAV Orbit Follower/1 -> Bus Creator/1  "LAP"

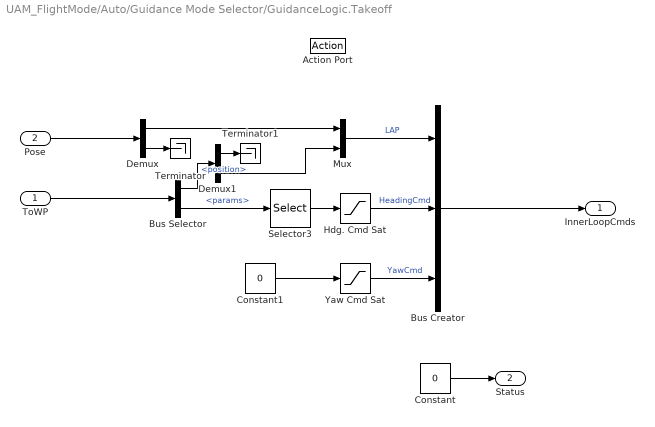
== system UAM_FlightMode/Auto/Guidance Mode Selector/GuidanceLogic.Takeoff ==
  ToWP : Inport  OutDataTypeStr=Bus: UAVPathManagerBus
  Pose : Inport  Port=2
  Action Port : ActionPort
      settings: CopyFcn=Stateflow.SLINSF.SimulinkMan.removeBlockPreDeleteFcn  PreDeleteFcn=Stateflow.SLINSF.SimulinkMan.unsafePredeleteFcn
  Bus Creator : BusCreator  Inputs=3  OutDataTypeStr=Bus: innerLoopCmdsBus  NonVirtualBus=on
      settings: InheritFromInputs=off
  Bus Selector : BusSelector  OutputSignals=position,params
  Constant : Constant  Value=0  OutDataTypeStr=uint8
  Constant1 : Constant  Value=0
  Demux : Demux  Outputs=[2 2]
  Demux1 : Demux  Outputs=[2 1]
  Hdg. Cmd Sat : Saturate  UpperLimit=pi  LowerLimit=-pi
      settings: AttributesFormatString=[%<UpperLimit> %<LowerLimit>]
  Mux : Mux  Inputs=2
  Selector3 : Selector  InputPortWidth=4  IndexOptions=Index vector (dialog)  Indices=4  OutputSizes=1
  Terminator : Terminator
  Terminator1 : Terminator
  Yaw Cmd Sat : Saturate  UpperLimit=pi  LowerLimit=-pi
      settings: AttributesFormatString=[%<UpperLimit> %<LowerLimit>]
  InnerLoopCmds : Outport  OutDataTypeStr=Bus: innerLoopCmdsBus
  Status : Outport  Port=2
  wires:
  Hdg. Cmd Sat/1 -> Bus Creator/2  "HeadingCmd"
  Bus Creator/1 -> InnerLoopCmds/1
  Constant/1 -> Status/1
  Pose/1 -> Demux/1
  Yaw Cmd Sat/1 -> Bus Creator/3  "YawCmd"
  ToWP/1 -> Bus Selector/1
  Bus Selector/2 -> Selector3/1  "<params>"
  Demux/1 -> Mux/1
  Bus Selector/1 -> Demux1/1  "<position>"
  Demux/2 -> Terminator/1
  Demux1/1 -> Terminator1/1
  Selector3/1 -> Hdg. Cmd Sat/1
  Constant1/1 -> Yaw Cmd Sat/1
  Demux1/2 -> Mux/2
  Mux/1 -> Bus Creator/1  "LAP"

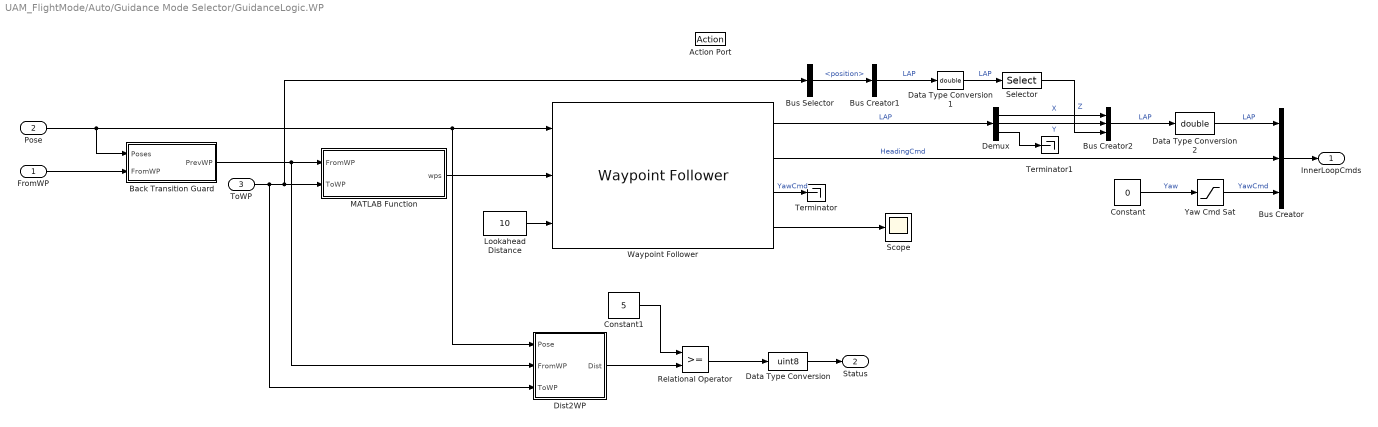
== system UAM_FlightMode/Auto/Guidance Mode Selector/GuidanceLogic.WP ==
  FromWP : Inport  OutDataTypeStr=Bus: UAVPathManagerBus
  Pose : Inport  Port=2
  ToWP : Inport  Port=3  OutDataTypeStr=Bus: UAVPathManagerBus
  Action Port : ActionPort
      settings: CopyFcn=Stateflow.SLINSF.SimulinkMan.removeBlockPreDeleteFcn  PreDeleteFcn=Stateflow.SLINSF.SimulinkMan.unsafePredeleteFcn
  Back Transition Guard : Subsystem
  Bus Creator : BusCreator  Inputs=3  OutDataTypeStr=Bus: innerLoopCmdsBus  NonVirtualBus=on
  Bus Creator1 : BusCreator  Inputs=1
  Bus Creator2 : BusCreator  Inputs=3
  Bus Selector : BusSelector  OutputSignals=position
  Constant : Constant  Value=0  OutDataTypeStr=double
  Constant1 : Constant  Value=5
  Data Type Conversion : DataTypeConversion  OutDataTypeStr=uint8  SaturateOnIntegerOverflow=off  RndMeth=Floor
  Data Type Conversion1 : DataTypeConversion  OutDataTypeStr=double  SaturateOnIntegerOverflow=off  RndMeth=Floor
  Data Type Conversion2 : DataTypeConversion  OutDataTypeStr=double  SaturateOnIntegerOverflow=off  RndMeth=Floor
  Demux : Demux  Outputs=3
  Dist2WP : Subsystem
  Lookahead Distance : Constant  Value=10  OutDataTypeStr=double
  MATLAB Function : MATLAB Function  TreatAsAtomicUnit=on
  Relational Operator : RelationalOperator  OutDataTypeStr=boolean  RndMeth=Simplest  InputSameDT=off
  Scope : Scope
  Selector : Selector  InputPortWidth=3  IndexOptions=Index vector (dialog)  Indices=3  OutputSizes=1
  Terminator : Terminator
  Terminator1 : Terminator
  Waypoint Follower : uavalgslib/Waypoint Follower  UAVType=multirotor  StartFrom=closest  TransitionRadiusSource=internal  TransitionRadius=R_WAYPOINTTRANSITION  MinLookaheadDistance=0.1  HoverAtLastWaypoint=off  YawInput=on  ShowCrossTrackErrorOutput=off  ShowStatusOutput=off  SimulateUsing=Code generation
  Yaw Cmd Sat : Saturate  UpperLimit=pi  LowerLimit=-pi
      settings: AttributesFormatString=[%<UpperLimit> %<LowerLimit>]
  InnerLoopCmds : Outport  OutDataTypeStr=Bus: innerLoopCmdsBus
  Status : Outport  Port=2
  wires:
  Data Type Conversion/1 -> Status/1
  Bus Creator/1 -> InnerLoopCmds/1
  ToWP/1 -> Dist2WP/3(ToWP), Bus Selector/1, MATLAB Function/2(ToWP)
  MATLAB Function/1(wps) -> Waypoint Follower/2
  Waypoint Follower/2 -> Bus Creator/2  "HeadingCmd"
  Waypoint Follower/4 -> Scope/1
  Dist2WP/1(Dist) -> Relational Operator/2
  FromWP/1 -> Back Transition Guard/2(FromWP)
  Relational Operator/1 -> Data Type Conversion/1
  Back Transition Guard/1(PrevWP) -> Dist2WP/2(FromWP), MATLAB Function/1(FromWP)
  Pose/1 -> Back Transition Guard/1(Poses), Waypoint Follower/1, Dist2WP/1(Pose)
  Lookahead Distance/1 -> Waypoint Follower/3
  Waypoint Follower/3 -> Terminator/1  "YawCmd"
  Constant/1 -> Yaw Cmd Sat/1  "Yaw"
  Yaw Cmd Sat/1 -> Bus Creator/3  "YawCmd"
  Constant1/1 -> Relational Operator/1
  Bus Creator1/1 -> Data Type Conversion1/1  "LAP"
  Waypoint Follower/1 -> Demux/1  "LAP"
  Demux/3 -> Terminator1/1
  Data Type Conversion1/1 -> Selector/1  "LAP"
  Selector/1 -> Bus Creator2/3  "Z"
  Demux/1 -> Bus Creator2/1  "X"
  Demux/2 -> Bus Creator2/2  "Y"
  Bus Creator2/1 -> Data Type Conversion2/1  "LAP"
  Data Type Conversion2/1 -> Bus Creator/1  "LAP"
  Bus Selector/1 -> Bus Creator1/1  "<position>"

== system UAM_FlightMode/Auto/Guidance Mode Selector/GuidanceLogic.WP/Back Transition Guard ==
  note: Set previous waypoint to current location if the UAV has just exited back transition
  Poses : Inport
  FromWP : Inport  Port=2
  Bus Selector : BusSelector  OutputSignals=mode
  Bus Selector1 : BusSelector  OutputSignals=position,params,mode
  Constant : Constant  Value=6
  Equal : RelationalOperator  Operator===  OutDataTypeStr=boolean  RndMeth=Simplest  InputSameDT=off
  Switch : Switch  Criteria=u2 > Threshold  SaturateOnIntegerOverflow=off  InputSameDT=off
  Triggered Subsystem : Subsystem  TreatAsAtomicUnit=on
  Out Bus Element2 : Outport  PortName=PrevWP  Element=mode
  Out Bus Element : Outport  PortName=PrevWP  Element=position
  Out Bus Element1 : Outport  PortName=PrevWP  Element=params
  wires:
  FromWP/1 -> Bus Selector1/1, Bus Selector/1
  Bus Selector/1 -> Equal/2  "<mode>"
  Constant/1 -> Equal/1
  Equal/1 -> Switch/2, Triggered Subsystem/Trigger
  Poses/1 -> Triggered Subsystem/1(Poses)
  Triggered Subsystem/1(HoldPositionValue) -> Switch/1
  Switch/1 -> Out Bus Element/1
  Bus Selector1/2 -> Out Bus Element1/1  "<params>"
  Bus Selector1/3 -> Out Bus Element2/1  "<mode>"
  Bus Selector1/1 -> Switch/3  "<position>"

== system UAM_FlightMode/Auto/Guidance Mode Selector/GuidanceLogic.WP/Dist2WP ==
  Pose : Inport
  FromWP : Inport  Port=2
  ToWP : Inport  Port=3
  Bus Selector : BusSelector  OutputSignals=position
  Bus Selector1 : BusSelector  OutputSignals=position
  Demux : Demux  Outputs=[3 1]
  Dot Product : DotProduct  OutDataTypeStr=Inherit: Inherit via internal rule
  Subsystem : Subsystem
  Sum : Sum  Inputs=|-+
  Sum1 : Sum  Inputs=|+-
  Terminator : Terminator
  Dist : Outport
  wires:
  Sum1/1 -> Subsystem/1(V)
  Demux/2 -> Terminator/1
  Bus Selector/1 -> Sum/2, Sum1/1  "<position>"
  Demux/1 -> Sum/1
  Bus Selector1/1 -> Sum1/2  "<position>"
  Sum/1 -> Dot Product/1
  Subsystem/1(V_unit) -> Dot Product/2
  Pose/1 -> Demux/1
  Dot Product/1 -> Dist/1
  ToWP/1 -> Bus Selector/1
  FromWP/1 -> Bus Selector1/1

== system UAM_FlightMode/Auto/Guidance Mode Selector/GuidanceLogic.WP/Back Transition Guard/Triggered Subsystem ==
  Poses : Inport
  Trigger : TriggerPort  VariantControl=(inherit)
  Reshape : Reshape  OutputDimensionality=Customize  OutputDimensions=[3,1]
  Selector : Selector  InputPortWidth=4  IndexOptions=Index vector (dialog)  Indices=[1 2 3]  OutputSizes=1
  HoldPositionValue : Outport
  wires:
  Poses/1 -> Selector/1
  Selector/1 -> Reshape/1
  Reshape/1 -> HoldPositionValue/1

== system UAM_FlightMode/Auto/Guidance Mode Selector/GuidanceLogic.WP/Dist2WP/Subsystem ==
  V : Inport
  Dot Product1 : DotProduct  OutDataTypeStr=Inherit: Inherit via internal rule
  Product : Product  Inputs=*/
  Saturation : Saturate  UpperLimit=inf  LowerLimit=0.00001
  Sqrt : Sqrt
  V_unit : Outport
  wires:
  V/1 -> Dot Product1/2, Dot Product1/1, Product/1
  Sqrt/1 -> Product/2
  Dot Product1/1 -> Saturation/1
  Saturation/1 -> Sqrt/1
  Product/1 -> V_unit/1

== stateflow chart UAM_FlightMode/Manual/Basic Control  Switching ==
  state STATE_MACHINE
    state Transition
      en:
      flightMode = flightState.Transition;
      controlMode.inTransition = 1;
      controlMode.TransitionCondition = 0;
    state HOVER
      en:
      flightMode = flightState.Hover;
    state FWCOMPLETE
      en:
      controlMode.TransitionCondition=1;
      flightMode = flightState.FixedWing;
    state Start
      en:
      flightMode=PresetMode;
      %conrtolmode
      controlMode.lateralGuidance = 0;
      controlMode.airspeedAltitude = 0;
      controlMode.attitude = 0;
      controlMode.manual = 1;
      controlMode.armed = 0;
      controlMode.inTransition = 0;
      controlMode.TransitionCondition = 0;
      controlMode.BackTransitionCondition = 0;
    state FixedWing
      en:
      flightMode = flightState.FixedWing;
      controlMode.attitude = 1;
      controlMode.inTransition = 0;
      controlMode.TransitionCondition = 1;
    state BackTransition
      en:
      flightMode = flightState.BackTransition;
      controlMode.inTransition = 1;
      controlMode.BackTransitionCondition = 0;
    state HVCOMPLETE
      en:
      controlMode.inTransition = 0;
      controlMode.BackTransitionCondition = 1;
      flightMode = flightState.Hover;
    (default) -> Start
    (junction 54) -> HOVER [order 1] : [trigger(5) < 1500 && flightMode == flightState.Hover ]
    HOVER -> Transition : [trigger(5) >= 1500 && flightMode == flightState.Hover]
    Transition -> FWCOMPLETE : [transitionConditionMet(a, Vt)]
    Start -> (junction 54)
    (junction 54) -> FixedWing [order 2] : [trigger(5) >= 1500 && flightMode == flightState.FixedWing]
    FixedWing -> BackTransition : [trigger(5) < 1500 && flightMode == flightState.FixedWing]
    BackTransition -> HVCOMPLETE : [backConditionMet(a, States)]
  data: alpha function_input double size=1; valid function_output; Vtransition function_input; alpha function_input; states function_input Bus: GuidanceStates; valid function_output; controlMode output Bus: controlMode; PresetMode input; States input; trigger input; Vt parameter double; a input size=1; flightMode output
  function valid = transitionConditionMet(alpha, Vtransition):
    | %function valid=transitionConditionMet(TransitionStates,Vtransition)
    | %wingsLevel
    | %if((States.Tilt>=1.57)&&(vecnorm(States.Ve)>Vt))
    | %   valid=true;
    | %else
    | %    valid=false;
    | %end
    | %end
    | 
    | function valid = transitionConditionMet(alpha, Vtransition)
    |     if (alpha >= 1.0) && (vecnorm(States.Ve) > Vtransition)
    |         valid = true;
    |     else
    |         valid = false;
    |     end
    | end
  function valid = backConditionMet(alpha, states):
    | function valid = backConditionMet(alpha, states)
    |     if ( alpha <= 0.01 ) && ( abs(states.Ve(1)) < 4.0 )
    |         valid = true;
    |     else
    |         valid = false;
    |     end
    | end

== stateflow chart UAM_FlightMode/Emergency/Basic Control  Switching ==
  state STATE_MACHINE
    state Transition
      en:
      flightMode = flightState.Transition;
      controlMode.inTransition = 1;
      controlMode.TransitionCondition = 0;
    state HOVER
      en:
      flightMode = flightState.Hover;
    state FWCOMPLETE
      en:
      controlMode.TransitionCondition=1;
      flightMode = flightState.FixedWing;
    state Start
      en:
      flightMode=PresetMode;
      %conrtolmode
      controlMode.lateralGuidance = 0;
      controlMode.airspeedAltitude = 0;
      controlMode.attitude = 0;
      controlMode.manual = 1;
      controlMode.armed = 0;
      controlMode.inTransition = 0;
      controlMode.TransitionCondition = 0;
      controlMode.BackTransitionCondition = 0;
    state FixedWing
      en:
      flightMode = flightState.FixedWing;
      controlMode.attitude = 1;
      controlMode.inTransition = 0;
      controlMode.TransitionCondition = 1;
    state BackTransition
      en:
      flightMode = flightState.BackTransition;
      controlMode.inTransition = 1;
      controlMode.BackTransitionCondition = 0;
    state HVCOMPLETE
      en:
      controlMode.inTransition = 0;
      controlMode.BackTransitionCondition = 1;
      flightMode = flightState.Hover;
    (default) -> Start
    (junction 54) -> HOVER [order 1] : [trigger(5) < 1500 && flightMode == flightState.Hover ]
    HOVER -> Transition : [trigger(5) >= 1500 && flightMode == flightState.Hover]
    Transition -> FWCOMPLETE : [transitionConditionMet(a, Vt)]
    Start -> (junction 54)
    (junction 54) -> FixedWing [order 2] : [trigger(5) >= 1500 && flightMode == flightState.FixedWing]
    FixedWing -> BackTransition : [trigger(5) < 1500 && flightMode == flightState.FixedWing]
    BackTransition -> HVCOMPLETE : [backConditionMet(a, States)]
  data: alpha function_input double size=1; valid function_output; Vtransition function_input; alpha function_input; states function_input Bus: GuidanceStates; valid function_output; controlMode output Bus: controlMode; PresetMode input; States input; trigger input; Vt parameter double; a input size=1; flightMode output
  function valid = transitionConditionMet(alpha, Vtransition):
    | %function valid=transitionConditionMet(TransitionStates,Vtransition)
    | %wingsLevel
    | %if((States.Tilt>=1.57)&&(vecnorm(States.Ve)>Vt))
    | %   valid=true;
    | %else
    | %    valid=false;
    | %end
    | %end
    | 
    | function valid = transitionConditionMet(alpha, Vtransition)
    |     if (alpha >= 1.0) && (vecnorm(States.Ve) > Vtransition)
    |         valid = true;
    |     else
    |         valid = false;
    |     end
    | end
  function valid = backConditionMet(alpha, states):
    | function valid = backConditionMet(alpha, states)
    |     if ( alpha <= 0.01 ) && ( abs(states.Ve(1)) < 4.0 )
    |         valid = true;
    |     else
    |         valid = false;
    |     end
    | end

== stateflow chart UAM_FlightMode/Auto/Guidance Mode Selector ==
  settings: updateMethod=DISCRETE  sampleTime=UAVSampleTime*4
  state GuidanceLogic
    state FIXED_WING_WAYPOINT
      en:
      controlMode.airspeedAltitude = 1;
      controlMode.attitude = 1;
      controlMode.lateralGuidance = 1;
      state WAYPOINT
    state FIXED_WING_ENTRY
      state Stabilize
        en:
        FlightMode=flightState.FixedWing;
        controlMode.attitude = 1;
        controlMode.airspeedAltitude = 0;
        controlMode.lateralGuidance = 0;
        %Transition once done.
        FixedWingSP.yaw = 0;
        FixedWingSP.pitch = 0;
        FixedWingSP.roll = 0;
        FixedWingSP.airspeed=14;
        Status= uint8(0);
      state FIXEDWINGFLIGHT
        en:
        % Control mode
        controlMode.airspeedAltitude = 1;
        controlMode.attitude = 1;
        controlMode.lateralGuidance = 1;
        % Setpoint init
        aacSP.L1 = 25;
        aacSP.airspeed = 14;
        aacSP.altitude = 0;
        aacSP.course=0;
      (default) -> Stabilize
      Stabilize -> FIXEDWINGFLIGHT : after(0.5,sec)
    state Start
      en:
      %Set Flight mode to hover
      FlightMode=PresetMode;
      %Set default settings
      % Control mode
      controlMode.airspeedAltitude = 1;
      controlMode.attitude = 1;
      controlMode.lateralGuidance = 0;
      controlMode.TransitionCondition = 0;
      controlMode.BackTransitionCondition=0;
      controlMode.land = 1;
      % Setpoint init
      FixedWingSP.yaw = 0;
      FixedWingSP.pitch = 0;
      FixedWingSP.roll = 0;
      FixedWingSP.airspeed=14;
      aacSP.L1 = 25;
      aacSP.airspeed = 14;
      aacSP.altitude = 0;
      aacSP.course=0;
      InnerLoopCmds.YawCmd=0;
    state FIXED_WING_ORBIT
      en:
      controlMode.airspeedAltitude = 1;
      controlMode.attitude = 1;
      controlMode.lateralGuidance = 1;
      state ORBIT
    state HOVER_ENTRY
      en:
      FlightMode=flightState.Hover;
      controlMode.inTransition=0;
    state Takeoff
    state WP
    state Orbit
    state PreTransition
      en:
      FlightMode=flightState.FixedWing;
      controlMode.airspeedAltitude = 1;
      controlMode.attitude = 1;
      controlMode.lateralGuidance = 1;
      % Setpoint init
      aacSP.L1 = 25;
      aacSP.airspeed = 14;
      aacSP.altitude = altitudeHold;
      aacSP.course=courseHold;
    state BackTransition
    state ForwardTransition
    state TransitionStep
      controlMode.TransitionStep=uint8(1);
    state FWCOMPLETE
      Status=uint8(1);
      controlMode.TransitionCondition=uint8(1);
    state BackCOMPLETE
      Status=uint8(1);
      controlMode.BackTransitionCondition=uint8(1)
    state Land
      state Descend
      state ToLand
      (default) -> ToLand
      ToLand -> Descend [order 1] : [(norm(Pose(1:2)-ToWP.position(1:2)) <= 30)]
    state Landcommand
      controlMode.land = 0;
    (default) -> Start
    Start -> (junction 5)
    FIXEDWINGFLIGHT -> WAYPOINT [order 2] : [(mode==2)]
        | {Status=uint8(0);}
    FIXEDWINGFLIGHT -> ORBIT [order 1] : [(mode==3)]
        | {Status= uint8(0);}
    (junction 262) -> FIXED_WING_ENTRY
    (junction 5) -> FIXED_WING_ORBIT [order 6] : [(mode==3)&&(FlightMode==flightState.FixedWing)]
        | {Status=uint8(0);}
    (junction 5) -> (junction 262) [order 3] : [(FlightMode==flightState.Transition)]
        | {controlMode.inTransition=0;}
    (junction 255) -> HOVER_ENTRY
    (junction 5) -> (junction 255) [order 4] : [(FlightMode==flightState.BackTransition)]
        | {controlMode.inTransition=0;}
    HOVER_ENTRY -> (junction 12)
    (junction 257) -> FIXED_WING_WAYPOINT
    Takeoff -> WP : [Pose(3) <= ToWP.position(3)]{Status = uint8(1);}
    GuidanceLogic -> (junction 5) : [(hasChanged(mode))]
    (junction 5) -> Takeoff [order 5] : [(mode == 1)&&(FlightMode==flightState.Hover)]
        | {controlMode.inTransition=0;}
    (junction 5) -> (junction 257) [order 2] : [(mode==2)&&(FlightMode==flightState.FixedWing)]
        | {Status=uint8(0);}
    (junction 5) -> (junction 260) [order 1] : [(mode==6)&&(FlightMode==flightState.FixedWing)]
        | {courseHold=States.course;
        | altitudeHold=-States.Xe(3); }
    (junction 5) -> (junction 12) [order 7] : [FlightMode==flightState.Hover]
        | {controlMode.inTransition=0;}
    (junction 260) -> PreTransition
    (junction 12) -> WP [order 1] : [(mode==2)]
    (junction 12) -> (junction 17) [order 2]
    (junction 17) -> Orbit [order 1] : [(mode==3)]
    (junction 17) -> (junction 22) [order 2]
    PreTransition -> BackTransition : after(5,sec)
        | {FlightMode=flightState.BackTransition;
        | controlMode.inTransition=1;
        | controlMode.BackTransitionCondition = 0;}
    BackTransition -> BackCOMPLETE : [backConditioMet(States, a)]
    (junction 22) -> ForwardTransition [order 1] : [(mode==6)]
        | {FlightMode=flightState.Transition;
        | controlMode.inTransition=1;
        | controlMode.TransitionCondition=uint8(0);
        |
        | }
    (junction 22) -> Land [order 2]
    TransitionStep -> FWCOMPLETE : [transitionConditionMet(a)]
    ForwardTransition -> TransitionStep : [transitionStepConditionMet(a)]
    ToLand -> Landcommand [order 2] : [States.Ve(3) >= -0.000001 && duration(States.Ve(3) >= -0.000001) > 8]
  note: [(mode==4)]
  (default) -> GuidanceLogic
  data: sf_internal_action_state_placeholder_data local double size=1 =0; sf_internal_action_state_placeholder_data local double size=1 =0; sf_internal_action_state_placeholder_data local double size=1 =0; sf_internal_action_state_placeholder_data local double size=1 =0; sf_internal_action_state_placeholder_data local double size=1 =0; sf_internal_action_state_placeholder_data local double size=1 =0; sf_internal_action_state_placeholder_data local double size=1 =0; sf_internal_action_state_placeholder_data local double size=1 =0; sf_internal_action_state_placeholder_data local double size=1 =0; states function_input; alpha function_input double; valid function_output; alpha function_input double; valid function_output; alpha function_input double; valid function_output; mode input; ToWP input Bus: UAVPathManagerBus; Status output uint8; FromWP input Bus: UAVPathManagerBus; Pose input; GdncMode output Enum: GdncModeType; States input; aacSP output Bus: AAC; FixedWingSP output Bus: FixedWingCommandBus; controlMode output Bus: controlMode; FlightMode output; PresetMode input; courseHold local; altitudeHold local; Vt parameter double; InnerLoopCmds output Bus: innerLoopCmdsBus; zGround parameter; Ground input; a input
  function valid = backConditioMet(states, alpha):
    | function valid = backConditioMet(states, alpha)
    | %( abs(states.Ve(1)) < 4.0 ) && 
    | if  ( alpha <= 0.01 )
    |     valid = true;
    | else
    |     valid = false;
    | end
    | end
  function valid = transitionStepConditionMet(alpha):
    | %function valid=transitionConditionMet(TransitionSt,Vtransition)
    | %wingsLevel
    | %if(States.Tilt>=1.57)&&(vecnorm(States.Ve)>Vt)
    | %   valid=true;
    | %else
    | %    valid=false;
    | %end
    | %end
    | 
    | function valid = transitionStepConditionMet(alpha)
    | if (alpha >= 1.0) %&& (vecnorm(States.Ve) > Vtransition)
    |     valid = true;
    | else
    |     valid = false;
    | end
    | end
  function valid = transitionConditionMet(alpha):
    | %function valid=transitionConditionMet(TransitionSt,Vtransition)
    | %wingsLevel
    | %if(States.Tilt>=1.57)&&(vecnorm(States.Ve)>Vt)
    | %   valid=true;
    | %else
    | %    valid=false;
    | %end
    | %end
    | 
    | function valid = transitionConditionMet(alpha)
    | if (alpha >= 1.0) %&& (vecnorm(States.Ve) > Vtransition)
    |     valid = true;
    | else
    |     valid = false;
    | end
    | end

== matlab function UAM_FlightMode/Auto/Guidance Mode Selector/GuidanceLogic.FIXED_WING_WAYPOINT.WAYPOINT/MATLAB Function ==
  data: toWP input; wps output; fromWP input; alt output
function [wps, alt]= fcn(toWP, fromWP)
    wps = zeros(2,3); %#ok<PREALL> 
    wps = [fromWP'; toWP'];
    alt = -toWP(3);
end

== matlab function UAM_FlightMode/Auto/Guidance Mode Selector/GuidanceLogic.Land.Descend/MATLAB Function ==
  data: FromWP input Bus: UAVPathManagerBus size=1; wps output; ToWPPos input size=[3 1]; ToWPParam input size=[4 1]
function wps = getLandingWaypoint(FromWP, ToWPPos, ToWPParam)

persistent outWPS

if isempty(outWPS)
    outWPS = double(zeros(2,4));
end

outWPS(1,:) = [FromWP.position' FromWP.params(4)];
outWPS(2,:) = [reshape(ToWPPos,1,[]), ToWPParam(4)];

wps = outWPS;

== matlab function UAM_FlightMode/Auto/Guidance Mode Selector/GuidanceLogic.Land.ToLand/MATLAB Function ==
  data: FromWP input Bus: UAVPathManagerBus size=1; wps output; ToWP input Bus: UAVPathManagerBus size=1
function wps = getLandingWaypoint(FromWP, ToWP)

persistent outWPS

if isempty(outWPS)
    outWPS = double(zeros(2,4));
end

outWPS(1,:) = [FromWP.position' FromWP.params(4)];
outWPS(2,:) = [ToWP.position(1:2)' FromWP.position(3) ToWP.params(4)];

wps = outWPS;

== matlab function UAM_FlightMode/Auto/Guidance Mode Selector/GuidanceLogic.WP/MATLAB Function ==
  data: FromWP input Bus: UAVPathManagerBus size=1; wps output; ToWP input Bus: UAVPathManagerBus size=1
function wps = getWaypointMission(FromWP, ToWP)

persistent outWPS

if isempty(outWPS)
    outWPS = double(zeros(2,4));
end

outWPS(1,:) = [FromWP.position' FromWP.params(4)];
outWPS(2,:) = [ToWP.position' ToWP.params(4)];

wps = outWPS;

== matlab function UAM_FlightMode/Auto/Guidance Mode Selector/GuidanceLogic.FIXED_WING_WAYPOINT.WAYPOINT/MATLAB Function1 ==
  data: wp_in input; wp_out output
function wp_out = swapXY(wp_in)
% wp_in: [n x 3] 배열 (North, East, Alt)
% wp_out: [n x 3] 배열 (East, North, Alt)

    wp_out = wp_in;
    wp_out(:,1) = wp_in(:,2);  % East → col 1
    wp_out(:,2) = wp_in(:,1);  % North → col 2
end

== matlab function UAM_FlightMode/Auto/Guidance Mode Selector/GuidanceLogic.FIXED_WING_WAYPOINT.WAYPOINT/MATLAB Function2 ==
  data: pose_in input; pose_out output
function pose_out = swapPoseXY(pose_in)
% pose_in: [1x4] (x, y, z, yaw)
% pose_out: [1x4] (y, x, z, yaw)

    pose_out = pose_in;
    pose_out(1) = pose_in(2);  % x ← y
    pose_out(2) = pose_in(1);  % y ← x
end

== matlab function UAM_FlightMode/Auto/Guidance Mode Selector/GuidanceLogic.ForwardTransition/MATLAB Function ==
  data: toWP input; wps output; fromWP input; alt output
function [wps, alt]= fcn(toWP, fromWP)
    wps = zeros(2,3); %#ok<PREALL> 
    wps = [fromWP'; toWP'];
    alt = -toWP(3);
end
